simulink model "Decremental_Counter"  (R2021a)
settings: Solver=VariableStepAuto  StartTime=0.0  StopTime=10.0  RelTol=1e-3
settings Model: Creator=Moamen_Hamed  LastModifiedBy=Mahmoud Shams El-Din

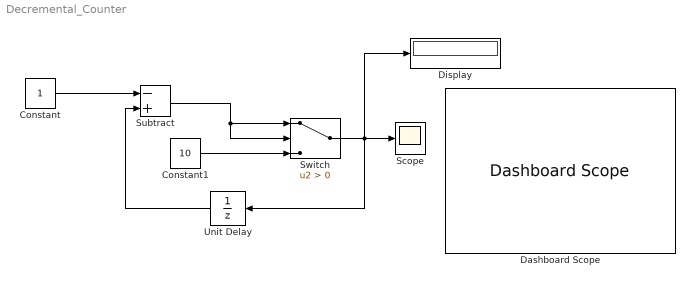
== system Decremental_Counter ==
  Constant : Constant
  Constant1 : Constant  Value=10
  Dashboard Scope : DashboardScope
  Display : Display
  Scope : Scope
  Subtract : Sum  Inputs=-+
  Switch : Switch  Criteria=u2 > Threshold
  Unit Delay : UnitDelay  InitialCondition=11  SampleTime=-1  HasFrameUpgradeWarning=on
  wires:
  Constant/1 -> Subtract/1
  Unit Delay/1 -> Subtract/2
  Switch/1 -> Scope/1, Unit Delay/1, Display/1
  Subtract/1 -> Switch/2, Switch/1
  Constant1/1 -> Switch/3
